simulink model "BuckBoost"  (R2019a)
settings: Solver=FixedStepDiscrete  StartTime=0.0  StopTime=0.1  RelTol=1e-3
libraries: powerlib x13, simulink x1, eePwmGenerator x1
settings Model: Creator=ryusl  LastModifiedBy=ryusl

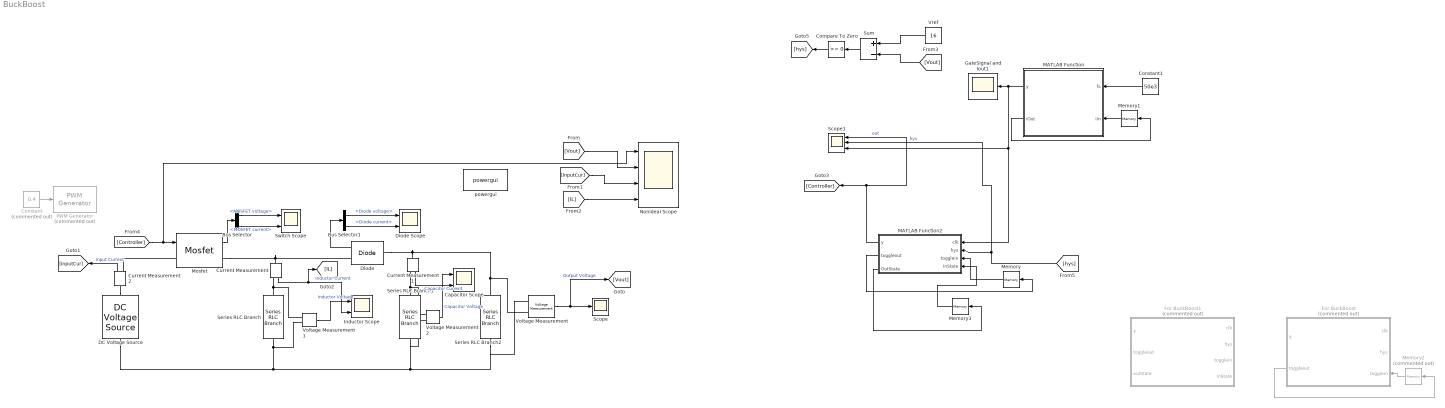
== system BuckBoost ==
  Bus Selector : BusSelector  OutputSignals=MOSFET voltage,MOSFET current
  Bus Selector1 : BusSelector  OutputSignals=Diode voltage,Diode current
  Capacitor Scope : Scope  NumInputPorts=2
  Compare To Zero : simulink/Logic and Bit Operations/Compare To Zero  relop=>=  OutDataTypeStr=boolean
  Constant : Constant  Commented=on  Value=0.4
  Constant1 : Constant  Value=50e3  SampleTime=1e-6
  Current Measurement : powerlib/Measurements/Current Measurement  PhasorSimulation=off  OutputType=Complex  PSBequivalent=0
      settings: SourceProductName=Simscape Electrical
  Current Measurement1 : powerlib/Measurements/Current Measurement  PhasorSimulation=off  OutputType=Complex  PSBequivalent=0
      settings: SourceProductName=Simscape Electrical
  Current Measurement2 : powerlib/Measurements/Current Measurement  PhasorSimulation=off  OutputType=Complex  PSBequivalent=0
      settings: SourceProductName=Simscape Electrical
  DC Voltage Source : powerlib/Electrical Sources/DC Voltage Source  Amplitude=24  Measurements=None
      settings: SourceProductName=Simscape Electrical
  Diode : powerlib/Power Electronics/Diode  Ron=0.001  Lon=0  Vf=0  IC=0  UseSnubber=0  Rs=500  Cs=250e-9  Measurements=on
      settings: SourceProductName=Simscape Electrical
  Diode Scope : Scope  NumInputPorts=2
  For BuckBoost : MATLAB Function  Commented=on  TreatAsAtomicUnit=on
  For BuckBoost1 : MATLAB Function  Commented=on  TreatAsAtomicUnit=on
  GateSignal and Iout1 : Scope
  Inductor Scope : Scope  NumInputPorts=2
  MATLAB Function : MATLAB Function  TreatAsAtomicUnit=on
  MATLAB Function2 : MATLAB Function  TreatAsAtomicUnit=on
  Memory : Memory
  Memory1 : Memory
  Memory2 : Memory  Commented=on
  Memory3 : Memory
  Mosfet : powerlib/Power Electronics/Mosfet  Ron=0.001  Lon=0  Rd=0.0001  Vfd=0  IC=0  Rs=1e5  Cs=inf  Measurements=on
      settings: SourceProductName=Simscape Electrical
  Nonideal Scope : Scope  NumInputPorts=4
  PWM Generator : eePwmGenerator/PWM Generator  Commented=on  CarrCount=Up  Tper=1/(50e3)  Ts=1e-7
      settings: SourceProductName=Simscape Electrical
  Scope : Scope
  Scope1 : Scope  NumInputPorts=3
  Series RLC Branch : powerlib/Elements/Series RLC Branch  LConnTagsString=__new0  RConnTagsString=__new0  BranchType=RL  Resistance=105e-3  Inductance=0.68e-3  SetiL0=on  InitialCurrent=3  Capacitance=1e-6  Setx0=off  InitialVoltage=0  Measurements=None
      settings: SourceProductName=Simscape Electrical
  Series RLC Branch1 : powerlib/Elements/Series RLC Branch  LConnTagsString=__new0  RConnTagsString=__new0  BranchType=RC  Resistance=15e-3  Inductance=1e-3  SetiL0=off  InitialCurrent=0  Capacitance=100e-6  Setx0=on  InitialVoltage=-20  Measurements=None
      settings: SourceProductName=Simscape Electrical
  Series RLC Branch2 : powerlib/Elements/Series RLC Branch  LConnTagsString=__new0  RConnTagsString=__new0  BranchType=R  Resistance=8  Inductance=1e-3  SetiL0=off  InitialCurrent=0  Capacitance=50e-6  Setx0=off  InitialVoltage=0  Measurements=None
      settings: SourceProductName=Simscape Electrical
  Sum : Sum  Inputs=+|-
  Switch Scope : Scope  NumInputPorts=2
  Voltage Measurement : powerlib/Measurements/Voltage Measurement  PhasorSimulation=off  OutputType=Complex  PSBequivalent=0
      settings: SourceProductName=Simscape Electrical
  Voltage Measurement1 : powerlib/Measurements/Voltage Measurement  PhasorSimulation=off  OutputType=Complex  PSBequivalent=0
      settings: SourceProductName=Simscape Electrical
  Voltage Measurement2 : powerlib/Measurements/Voltage Measurement  PhasorSimulation=off  OutputType=Complex  PSBequivalent=0
      settings: SourceProductName=Simscape Electrical
  Vref : Constant  Value=16
  powergui : powerlib/powergui  Priority=1  SimulationMode=Discrete  SampleTime=1e-7  frequency=60  Iterations=50  frequencyindice=0  Pbase=100e6  ErrMax=1e-4  UnitsV=kV  UnitsW=MW  buscounter=0  FunctionMessages=off  echomessages=off  EnableUseOfTLC=off  CurrentSourceSwitches=off  DisableSnubberDevices=off  DisableRonSwitches=off  DisableVfSwitches=off  DisplayEquations=off  AutomaticDiscreteSolvers=off  SolverType=Tustin/Backward Euler (TBE)  Interpol=off  ExternalGateDelay=off  methode=off  Ts=100  x0status=blocks  SPID=on  SwTol=0  HookPort=off  NonlinearTolerance=0  nMaxIteration=15  ContinueOnMaxIteration=off  RestoreLinks=warning  ResistiveCurrentMeasurement=off  Frange=[0:2:500]  Ylog=off  Xlog=on  ShowGrid=off  save=off  variable=ZData  structure=0  ZoomFFT=off  StartTime=0.0  cycles=1  DisplayStyle=1  fundamental=60  FreqAxis=off  MaxFrequency=1000  frequencyindicesteady=1  RmsSteady=1  display=off
      settings: SourceProductName=Simscape Electrical
  wires:
  Constant/1 -> PWM Generator/1
  Voltage Measurement/1 -> [Vout], Scope/1  "Output Voltage"
  Current Measurement/1 -> [IL], Inductor Scope/2  "Inductor Current"
  Mosfet/1 -> Bus Selector/1
  Bus Selector/1 -> Switch Scope/1  "<MOSFET voltage>"
  Bus Selector/2 -> Switch Scope/2  "<MOSFET current>"
  Diode/1 -> Bus Selector1/1
  Bus Selector1/1 -> Diode Scope/1  "<Diode voltage>"
  Bus Selector1/2 -> Diode Scope/2  "<Diode current>"
  Voltage Measurement1/1 -> Inductor Scope/1  "Inductor Voltage"
  Voltage Measurement2/1 -> Capacitor Scope/1  "Capacitor Voltage"
  Current Measurement1/1 -> Capacitor Scope/2  "Capacitor Current"
  Current Measurement2/1 -> [InputCur]  "Input Current"
  [Vout] -> Nonideal Scope/2
  [InputCur] -> Nonideal Scope/3
  [IL] -> Nonideal Scope/4
  [hys] -> Scope1/2, MATLAB Function2/2(hys)  "hys"
  MATLAB Function/2(iOut) -> Memory1/1
  Memory1/1 -> MATLAB Function/2(iIn)
  MATLAB Function/1(y) -> Scope1/3, MATLAB Function2/1(clk), GateSignal and Iout1/1
  Sum/1 -> Compare To Zero/1
  MATLAB Function2/1(y) -> Scope1/1, [Controller]  "out"
  [Vout] -> Sum/2
  Vref/1 -> Sum/1
  MATLAB Function2/2(toggleout) -> Memory/1
  Constant1/1 -> MATLAB Function/1(fs)
  Memory/1 -> MATLAB Function2/3(togglein)
  Compare To Zero/1 -> [hys]
  [Controller] -> Nonideal Scope/1, Mosfet/1
  Memory2/1 -> For BuckBoost/3(togglein)
  For BuckBoost/2(toggleout) -> Memory2/1
  Memory3/1 -> MATLAB Function2/4(InState)
  MATLAB Function2/3(OutState) -> Memory3/1
  connections:
  Mosfet/RConn1 -- Current Measurement/LConn1 -- Diode/RConn1
  DC Voltage Source/LConn1 -- Voltage Measurement/LConn1 -- Series RLC Branch2/RConn1 -- Voltage Measurement2/LConn2 -- Series RLC Branch1/RConn1 -- Voltage Measurement1/LConn2 -- Series RLC Branch/RConn1
  Diode/LConn1 -- Current Measurement1/LConn1 -- Series RLC Branch2/LConn1 -- Voltage Measurement/LConn2
  Current Measurement/RConn1 -- Voltage Measurement1/LConn1 -- Series RLC Branch/LConn1
  Current Measurement1/RConn1 -- Voltage Measurement2/LConn1 -- Series RLC Branch1/LConn1
  Current Measurement2/LConn1 -- DC Voltage Source/RConn1
  Current Measurement2/RConn1 -- Mosfet/LConn1

== matlab function BuckBoost/For BuckBoost ==
  data: clk input; y output; hys input; togglein input; toggleout output
function [y,toggleout] = fcn(clk,hys,togglein)
if (clk == 1)
    if (hys == 1) %Vo is smaller, make gate signal off
        if (y == 1)
            y = 0;
            toggleout = 0;
        else
            y = 0;
            toggleout = 1;
        end
    else % (hys == 0) %Vo is higher, make gate signal on
        if (y == 1)
            y = 1;
            toggleout = 1;
        else
            y = 1;
            toggleout = 0;
        end
    end
else
    if (togglein == 1) % Still have a chance to switch
        if (hys == 1) % Vo is smaller, make gate signal off
            if (y == 1)
                y = 0;
                toggleout = 0;
            else
                y = 0;
                toggleout = 1;
            end
        else %Vo is higher, make gate signal on
            if (y == 1)
                y = 1;
                toggleout = 1;
            else
                y = 1;
                toggleout = 0;
            end
        end
    else
        if (y == 1)
            y = 1;
            toggleout = 0;
        else
            y = 0;
            toggleout = 0;
        end
    end
end
%     if (hys == 1)
%         if (togglein == 0)
%             y = 1;
%             toggleout = 0;
%         else
%             y = 0;
%             toggleout = 1;
%         end
%     else
%         y = 1;
%         toggleout = 0;
%     end
%end

== matlab function BuckBoost/MATLAB Function ==
  data: fs input; y output; iIn input; iOut output
function [y,iOut] = fcn(fs,iIn)
iOut = iIn;
cnt = (1/fs)/(1e-7);
cnt = int32(cnt); 
if (iIn >= cnt)
    iOut = 0;
    y = 0;
else
    if (iIn <= 2)
        y = 1;
        iOut = iOut + 1;
    else
        y = 0;
        iOut = iOut + 1;
    end
end

== matlab function BuckBoost/For BuckBoost1 ==
  data: clk input; y output; hys input; togglein input; toggleout output; inState input; outState output
function [y,toggleout,outState] = fcn(clk,hys,togglein,inState)
y = inState;
if (clk == 1)
    if (hys == 1) %Vo is smaller, make gate signal off
        if (y == 1)
            y = 0;
            toggleout = 0;
            outState = y;
        else
            y = 0;
            toggleout = 1;
            outState = y;
        end
    else % (hys == 0) %Vo is higher, make gate signal on
        if (y == 1)
            y = 1;
            toggleout = 1;
            outState = y;
        else
            y = 1;
            toggleout = 0;
            outState = y;
        end
    end
else
    if (togglein == 1) % Still have a chance to switch
        if (hys == 1) % Vo is smaller, make gate signal off
            if (y == 1)
                y = 0;
                toggleout = 0;
                outState = y;
            else
                y = 0;
                toggleout = 1;
                outState = y;
            end
        else %Vo is higher, make gate signal on
            if (y == 1)
                y = 1;
                toggleout = 1;
                outState = y;
            else
                y = 1;
                toggleout = 0;
                outState = y;
            end
        end
    else
        if (y == 1)
            y = 1;
            toggleout = 0;
            outState = y;
        else
            y = 0;
            toggleout = 0;
            outState = y;
        end
    end
end
%     if (hys == 1)
%         if (togglein == 0)
%             y = 1;
%             toggleout = 0;
%         else
%             y = 0;
%             toggleout = 1;
%         end
%     else
%         y = 1;
%         toggleout = 0;
%     end
%end

== matlab function BuckBoost/MATLAB Function2 ==
  data: clk input; y output; hys input; togglein input; toggleout output; InState input; OutState output
function [y,toggleout,OutState] = fcn(clk,hys,togglein,InState)
if (clk == 1)
    y = 1;
    OutState = y;
    toggleout = 1;
else
    if (togglein == 1) % Still have a bullet
        if (hys == 1) %Vo is smaller, make gate signal on
            y = 0;
            OutState = y;
            toggleout = 0;
        else
            y = 1;
            OutState = y;
            toggleout = 1;
        end
    else
        OutState = InState;
        y = InState
        toggleout = 0;
%         if (y == 1)
%             y = 1;
%         else
%             y = 0;
%         end
    end
end
%     if (hys == 1) %Vo is smaller, make gate signal on
%         if (togglein == 0)
%             y = 1;
%             toggleout = 0;
%         else
%             y = 0;
%             toggleout = 1;
%         end
%     else
%         y = 1;
%         toggleout = 0;
%     end
% end
